simulink model "plant_model"  (R2015b)
settings: Solver=ode45  StartTime=0.0  StopTime=10.0  RelTol=1e-3
values from neighbouring files (symbols this model uses):
  c = ureal('c',0.04,'Percentage',50)    [structured_uncertaines.m]
  delta_input = ultidyn('delta_input',[1 1],'Bound',1.0)    [unstructured_uncertaines.m]
  delta_output = ultidyn('delta_output',[1 1],'Bound',1.0)    [unstructured_uncertaines.m]
  k = ureal('k',4,'Percentage',50)    [structured_uncertaines.m]
  m = 1    [structured_uncertaines.m]
libraries: RCTblocks x4
settings Model: Creator=michele  LastModifiedBy=michele
settings DataIOCC: SaveFormat=Array
settings HardwareCC: ProdBitPerPointer=32  ProdLargestAtomicFloat=None  ProdIntDivRoundTo=Undefined  ProdEndianess=Unspecified  ProdWordSize=32  ProdHWDeviceType=32-bit Generic
settings GRTTargetCC: GeneratePreprocessorConditionals=Disable all
settings ConfigComp: CovModelRefEnable=Off  CovSFcnEnable=off

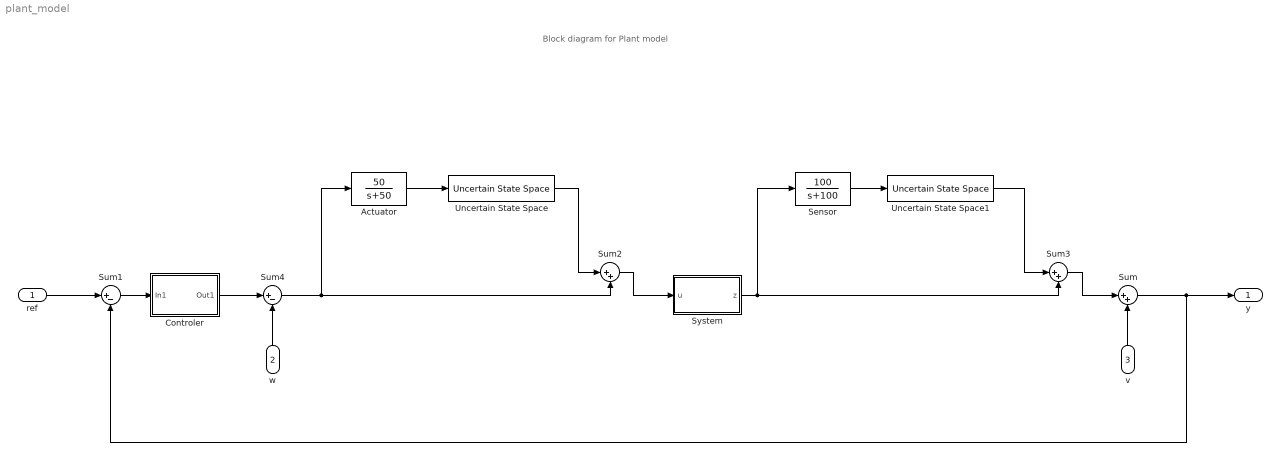
== system plant_model ==
  note: Block diagram for Plant model
  ref : Inport
  w : Inport  Port=2
  v : Inport  Port=3
  Actuator : TransferFcn  Numerator=[50]  Denominator=[1 50]
  Controler : Subsystem
  Sensor : TransferFcn  Numerator=[100]  Denominator=[1 100]
  Sum : Sum  Inputs=|++
  Sum1 : Sum  Inputs=|+-
  Sum2 : Sum  Inputs=|++
  Sum3 : Sum  Inputs=|++
  Sum4 : Sum  Inputs=|+-
  System : Subsystem
  Uncertain State Space : RCTblocks/Uncertain State Space  Tag=USS  USystem=ss(delta_input)  UValue=[]  X0=[]  uX0=[]
  Uncertain State Space1 : RCTblocks/Uncertain State Space  Tag=USS  USystem=ss(delta_output)  UValue=[]  X0=[]  uX0=[]
  y : Outport
  wires:
  Sum1/1 -> Controler/1(In1)
  Sum/1 -> Sum1/2, y/1
  v/1 -> Sum/2
  ref/1 -> Sum1/1
  Sum2/1 -> System/1(u)
  System/1(z) -> Sensor/1, Sum3/2
  Sum3/1 -> Sum/1
  Actuator/1 -> Uncertain State Space/1
  Uncertain State Space/1 -> Sum2/1
  Sensor/1 -> Uncertain State Space1/1
  Uncertain State Space1/1 -> Sum3/1
  Controler/1(Out1) -> Sum4/1
  Sum4/1 -> Sum2/2, Actuator/1
  w/1 -> Sum4/2

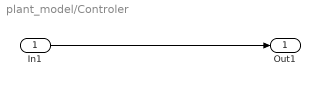
== system plant_model/Controler ==
  In1 : Inport
  Out1 : Outport
  wires:
  In1/1 -> Out1/1

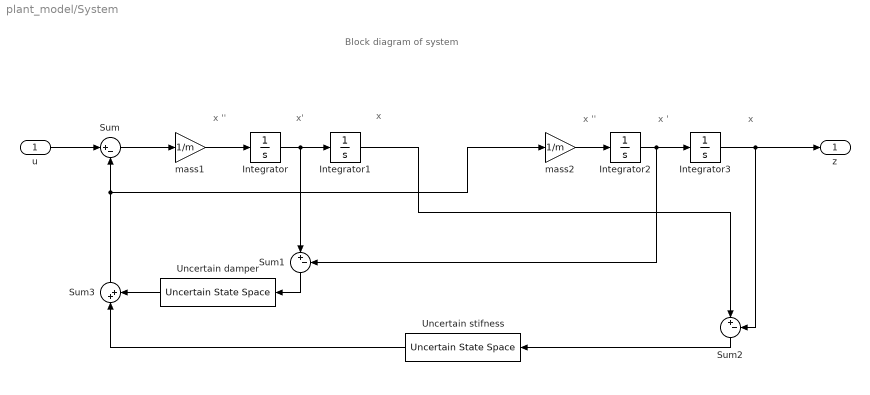
== system plant_model/System ==
  note: Block diagram of system
  note: x
  note: x'
  note: x ''
  note: x ''
  note: x '
  note: x
  u : Inport
  Integrator{,1..3} (4 alike) : Integrator
  Sum : Sum  Inputs=|+-
  Sum1 : Sum  Inputs=|+-
  Sum2 : Sum  Inputs=|+-
  Sum3 : Sum  Inputs=|++
  Uncertain damper : RCTblocks/Uncertain State Space  Tag=USS  USystem=ss(c)  UValue=[]  X0=[]  uX0=[]
  Uncertain stifness : RCTblocks/Uncertain State Space  Tag=USS  USystem=ss(k)  UValue=[]  X0=[]  uX0=[]
  mass1 : Gain  Gain=1/m
  mass2 : Gain  Gain=1/m
  z : Outport
  wires:
  Integrator/1 -> Sum1/1, Integrator1/1
  Integrator2/1 -> Sum1/2, Integrator3/1
  Sum1/1 -> Uncertain damper/1
  Integrator1/1 -> Sum2/1
  Integrator3/1 -> z/1, Sum2/2
  Sum2/1 -> Uncertain stifness/1
  Uncertain stifness/1 -> Sum3/1
  Sum3/1 -> Sum/2, mass2/1
  mass1/1 -> Integrator/1
  Sum/1 -> mass1/1
  mass2/1 -> Integrator2/1
  u/1 -> Sum/1
  Uncertain damper/1 -> Sum3/2
